simulink model "chap4_6sim"  (Simulink 3.00)
settings: Solver=ode45  StartTime=0.0  StopTime=10  RelTol=1e-3
settings Model: LastModifiedBy=liu

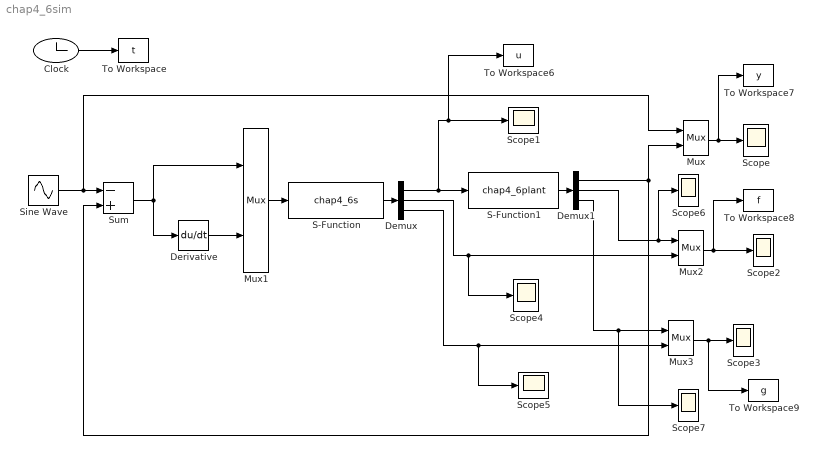
== system chap4_6sim ==
  Clock : Clock
  Demux : Demux  Outputs=3
  Demux1 : Demux  Outputs=3
  Derivative : Derivative
  Mux{,1..3} (4 alike) : Mux  Inputs=2
      settings: DisplayOption=none
  S-Function : S-Function  FunctionName=chap4_6s  PortCounts=[]  SFunctionModules=''
  S-Function1 : S-Function  FunctionName=chap4_6plant  PortCounts=[]  SFunctionModules=''
  Scope{,1..7} (8 alike) : Scope
      Scope settings: TimeRange=3  YMin=-0.1  YMax=-0.015  SaveToWorkspace=off  SaveName=ScopeData  MaxRows=500000
      Scope1 settings: TimeRange=3  YMin=-3  YMax=10  SaveToWorkspace=off  SaveName=ScopeData  MaxRows=500000
      Scope2 settings: TimeRange=3  YMin=-0.1  YMax=1  SaveToWorkspace=off  SaveName=ScopeData  MaxRows=500000
      Scope3 settings: TimeRange=3  YMin=-0.1  YMax=0.1  SaveToWorkspace=off  SaveName=ScopeData  MaxRows=500000
      Scope4 settings: TimeRange=3  YMin=-0.1  YMax=0.1  SaveToWorkspace=off  SaveName=ScopeData  MaxRows=500000
      Scope5 settings: TimeRange=3  YMin=-0.1  YMax=0.1  SaveToWorkspace=off  SaveName=ScopeData  MaxRows=500000
      Scope6 settings: TimeRange=3  YMin=-0.1  YMax=1  SaveToWorkspace=off  SaveName=ScopeData  MaxRows=500000
      Scope7 settings: TimeRange=3  YMin=-0.1  YMax=1  SaveToWorkspace=off  SaveName=ScopeData  MaxRows=500000
  Sine Wave : Sin  Amplitude=0.1  Frequency=pi  Phase=0  SampleTime=0
  Sum : Sum  Inputs=-+  SaturateOnIntegerOverflow=on
  To Workspace : ToWorkspace  VariableName=t  SampleTime=-1  SaveFormat=Matrix
  To Workspace6 : ToWorkspace  VariableName=u  SampleTime=-1  SaveFormat=Matrix
  To Workspace7 : ToWorkspace  VariableName=y  SampleTime=-1  SaveFormat=Matrix
  To Workspace8 : ToWorkspace  VariableName=f  SampleTime=-1  SaveFormat=Matrix
  To Workspace9 : ToWorkspace  VariableName=g  SampleTime=-1  SaveFormat=Matrix
  wires:
  Mux1/1 -> S-Function/1
  S-Function/1 -> Demux/1
  S-Function1/1 -> Demux1/1
  Demux1/1 -> Sum/2, Mux/2
  Sum/1 -> Mux1/1, Derivative/1
  Sine Wave/1 -> Sum/1, Mux/1
  Derivative/1 -> Mux1/2
  Demux/3 -> Scope5/1, Mux3/2
  Demux/2 -> Mux2/2, Scope4/1
  Demux/1 -> S-Function1/1, Scope1/1, To Workspace6/1
  Mux/1 -> Scope/1, To Workspace7/1
  Clock/1 -> To Workspace/1
  Mux2/1 -> Scope2/1, To Workspace8/1
  Mux3/1 -> Scope3/1, To Workspace9/1
  Demux1/2 -> Mux2/1, Scope6/1
  Demux1/3 -> Mux3/1, Scope7/1
